simulink model "Model"  (R2024b)
settings: Solver=VariableStepAuto  StartTime=0.0  StopTime=20  RelTol=1e-2
values from neighbouring files (symbols this model uses):
  camber = 1 *pi/180    (= 0.0174532925199)    [var.m]
  cgToRearAxle = 0.7    [var.m]
  cgVerticalToAxlePlane = 0.1    [var.m]
  lammux = 0.65    [var.m]
  lammuy = 0.65    [var.m]
  mass = 200    [var.m]
  maxBrakePressure = 5000000    [var.m]
  tirePressure = 83000    [var.m]
  tireRadius = 0.2057    [var.m]
  trackWidth = 1    [var.m]
  wheelAngleLimit = 45 *pi/180    (= 0.785398163397)    [var.m]
  yawPolarInertia = 200    [var.m]
undefined symbols (not defined in the file or in its folder): SteerLim, Ts, VEH
libraries: sim3dlib x4, autolibsharedcoupling x2, sim3dautolib x2, vehdynlibviscommon x2, simulink x1, autolibshared x1, autolibshareddiff x1, autolibmappedmotor x1, vehdynlibdriver x1, vehdynlibsteering x1, vehdynlibtire x1, vehdynlibsuspension x1
(part 1 of 3)
settings Model: Creator=owen  LastModifiedBy=owen

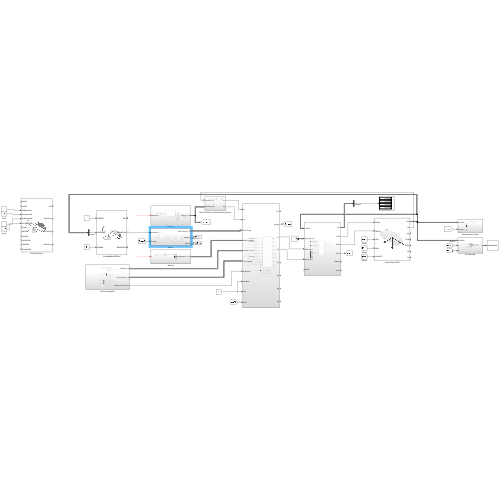
[thumbnail: Simulink's stored preview of the top-level diagram]
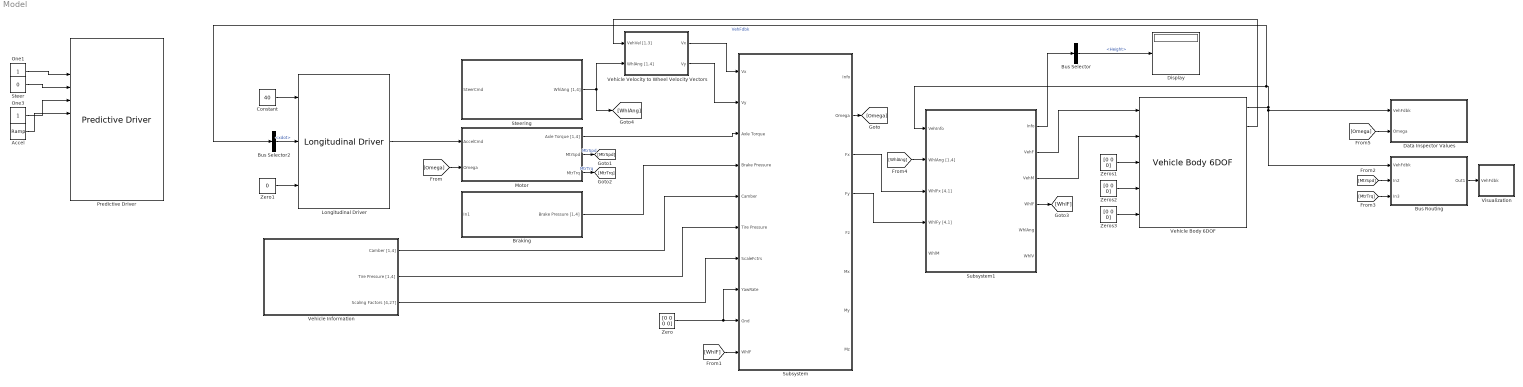
== system Model ==
  Accel : simulink/Sources/Ramp  slope=0.1  start=0  InitialOutput=0
  Braking : Subsystem
  Bus Selector : BusSelector  OutputSignals=Height
  Bus Selector2 : BusSelector  OutputSignals=BdyFrm.Cg.Vel.xdot
  Bus Routing : Subsystem
  Constant : Constant  Value=40
  Data Inspector Values : Subsystem
  Display : Display
  Longitudinal Driver : autolibshared/Longitudinal Driver  extAccelOvr=off  extDecelOvr=off  extAccelHld=off  extDecelHld=off  extAccelZero=off  extDecelZero=off  cntrlType=PI  shftType=None  velUnits=m/s  gearOut=off  Kp=10  Ki=5  Kff=.1  Kg=0  VehVelVec=[0 100]  KffVec=[.1 .1]  KpVec=[10 10]  KiVec=[5 5]  KgVec=[0 0]  m=1500  Kpt=3000  tau=.1  L=2  aR=200  bR=2.5  cR=.5  g=9.81  vnom=5  Kaw=1  tauerr=.01  tauPt=2  GearInit=0  tShift=.1  pdlVec=[0.1 0.4 0.5 0.9]  upShftTbl=[-1 12.9375 26.4375 39.9375 51.18749999999999 62.4375 72.84375 83.25;-1 16.3125 29.8125 43.3125 54.5624 65.8125 76.78125 87.75;-1 19.6875 33.1875 46.68749999999999 57.9375 69.1875 80.71875 92.25;-1 33 52.5 77.25 100.5 138.75 161.875 185]  dwnShftTbl=[1 9.5625 23.0625 36.5625 47.8125 59.0625 68.90625 78.75;1 12.9375 26.4375 39.9375 51.18749999999999 62.4375 72.84375 83.25;1 16.3125 29.8125 43.3125 54.562499 65.8125 76.78125 87.75;1 19.6875 33.1875 46.68749999999999 57.9375 69.1875 80.71875 92.25]  tClutch=.5  tRev=.5  tPark=120  aMode=2  UpGearVec="[0  1  2  3  4  5  6  7]"  DownGearVec="[1  2  3  4  5  6  7  8]"
      settings: LibrarySourceBlock=vehdynlibdriver/Longitudinal Driver
  Motor : Subsystem
  One1 : Constant  OutDataTypeStr=boolean
  One3 : Constant  OutDataTypeStr=boolean
  Predictive Driver : vehdynlibdriver/Predictive Driver  extAccelOvr=on  extDecelOvr=off  extAccelHld=off  extDecelHld=off  extAccelZero=off  extDecelZero=off  extSteerOvr=on  extSteerHld=off  extSteerZero=off  cntrlType=PI  cntrlTypeLat=Predictive  shftType=None  coordMode=SAE J670 (Z-down)  refType=Reference pose  velUnits=m/s  angUnits=rad  gearOut=off  steerOut=off  Kp=10  Ki=5  Kff=.1  Kg=0  VehVelVec=[0 100]  KffVec=[.1 .1]  KpVec=[10 10]  KiVec=[5 5]  KgVec=[0 0]  vnom=5  Kaw=1  tauerr=.01  tau=0.1  L=3  Kpt=3000  aR=200  bR=2.5  cR=.5  g=9.81  vecPose=off  dynamMode=off  PositionGainF=2.5  PositionGainR=2.5  YawRateGain=.2  DelayGain=.2  enableDrift=off  BetaRef=20*pi/180  KpBeta=1  KpDrift=2  KdDrift=1  KpPsi=6  KOmega=30  tOmega=1  a=cgToFrontAxle  b=cgToRearAxle  m=mass  Cy_f=cornerStiffness  Cy_r=cornerStiffness  I=yawPolarInertia  Ksteer=18  theta=wheelAngleLimit  Idl=3  Re=.3  lambda_mu=1  GearInit=0  tShift=.1  pdlVec=[0.1 0.4 0.5 0.9]  upShftTbl=[-1 12.9375 26.4375 39.9375 51.18749999999999 62.4375 72.84375 83.25;-1 16.3125 29.8125 43.3125 54.5624 65.8125 76.78125 87.75;-1 19.6875 33.1875 46.68749999999999 57.9375 69.1875 80.71875 92.25;-1 33 52.5 77.25 100.5 138.75 161.875 185]  dwnShftTbl=[-1 12.9375 26.4375 39.9375 51.18749999999999 62.4375 72.84375 83.25;-1 16.3125 29.8125 43.3125 54.5624 65.8125 76.78125 87.75;-1 19.6875 33.1875 46.68749999999999 57.9375 69.1875 80.71875 92.25;-1 33 52.5 77.25 100.5 138.75 161.875 185]  tClutch=.5  tRev=.5  tPark=120  UpGearVec="[0  1  2  3  4  5  6  7]"  DownGearVec="[1  2  3  4  5  6  7  8]"  aMode=2
  Steer : Constant  Value=0  OutDataTypeStr=Inherit: Inherit via back propagation
  Steering : Subsystem
  Subsystem : Subsystem
  Subsystem1 : Subsystem
  Vehicle Body 6DOF : vehdynlibeom/Vehicle Body 6DOF  extPos=on  extVel=on  extEuler=on  extRotRate=on  htchFMode=off  htchMMode=off  m=mass  a=cgToFrontAxle  b=cgToRearAxle  d=0  h=cgVerticalToAxlePlane  dh=1  hl=0  hh=0.1  Xe_o=[0,0, -0.25]  xbdot_o=[0,0,0]  eul_o=[0,0,0]  p_o=[0,0,0]  Iveh=[430 0 0; 0 1900 0; 0 0 2100]  w=[trackWidth,trackWidth]  z1m=0  z1R=[-.25,.125,.15]  z1I=[1.4,-.2,.1;-.2,1.4,.1;.1,.1,2.25].*0  z2m=0  z2R=[1.4,0,.8]  z2I=[1.4,-.2,.1;-.2,1.4,.1;.1,.1,2.25].*0  z3m=0  z3R=[.75,-.5,.4]  z3I=[5,-.1,-2;-2,9,.1;-.1,.1,6].*0  z4m=0  z4R=[.75,.5,.4]  z4I=[5,-.1,-2;-2,9,.1;-.1,.1,6].*0  z5m=0  z5R=[1.25,-.5,.4]  z5I=[5,-.1,-2;-2,9,.1;-.1,.1,6].*0  z6m=0  z6R=[1.25,-.5,.4]  z6I=[5,-.1,-2;-2,9,.1;-.1,.1,6].*0  z7m=0  z7R=[2,0,.25]  z7I=[1.4,-.2,.1;-.2,1.4,.1;.1,.1,2.25].*0  Af=longDragArea  Cd=longDragCoeff  Cl=longLiftCoeff  Cpm=.1  beta_w=[0:0.001:0.01]  Cs=[0:0.01:0.1]  Cym=[0:0.001:0.01]  Pabs=101325  extTamb=off  Tair=273  g=9.81  xdot_tol=.1  longOff=0  latOff=0  vertOff=0  wrapAng=on  aMode=2
  Vehicle Information : Subsystem
  Vehicle Velocity to Wheel Velocity Vectors : Subsystem
  Visualization : Subsystem
      mask Display: disp('Visualization')
  Zero : Constant  Value=[0 0 0 0]
  Zero1 : Constant  Value=0  OutDataTypeStr=Inherit: Inherit via back propagation
  Zeros1 : Constant  Value=[0 0 0]
  Zeros2 : Constant  Value=[0 0 0]
  Zeros3 : Constant  Value=[0 0 0]
  wires:
  ? -> Steering/1(SteerCmd)
  Steer/1 -> Predictive Driver/4
  One1/1 -> Predictive Driver/3
  Longitudinal Driver/2 -> Motor/1(AccelCmd)
  ? -> Braking/1(In1)
  Braking/1("Brake Pressure [1,4] ") -> Subsystem/4(Brake Pressure)
  Motor/1(Axle Torque [1,4]) -> Subsystem/3(Axle Torque)
  Vehicle Information/1(Camber [1,4]) -> Subsystem/5(Camber)
  Vehicle Information/2(Tire Pressure [1,4]) -> Subsystem/6(Tire Pressure)
  Vehicle Body 6DOF/2 -> Vehicle Velocity to Wheel Velocity Vectors/1(VehVel [1,3])
  Steering/1(WhlAng [1,4]) -> [WhlAng], Vehicle Velocity to Wheel Velocity Vectors/2(WhlAng [1,4])
  Vehicle Velocity to Wheel Velocity Vectors/2(Vy) -> Subsystem/2(Vy)
  Vehicle Velocity to Wheel Velocity Vectors/1(Vx) -> Subsystem/1(Vx)
  Vehicle Information/3(Scaling Factors [4,27]) -> Subsystem/7(ScaleFctrs)
  Subsystem/3(Fx) -> Subsystem1/3(WhlFx [4,1])
  Subsystem/4(Fy) -> Subsystem1/4(WhlFy [4,1])
  Subsystem1/2(VehF) -> Vehicle Body 6DOF/1
  Subsystem1/3(VehM) -> Vehicle Body 6DOF/2
  Zeros2/1 -> Vehicle Body 6DOF/4
  Zero/1 -> Subsystem/8(YawRate), Subsystem/9(Gnd)
  Vehicle Body 6DOF/1 -> Bus Routing/1(VehFdbk), Data Inspector Values/1(VehFdbk), Bus Selector2/1, Subsystem1/1(VehInfo)  "VehFdbk"
  Subsystem1/1(Info) -> Bus Selector/1
  Bus Selector/1 -> Display/1  "<Height>"
  Zeros1/1 -> Vehicle Body 6DOF/3
  Zeros3/1 -> Vehicle Body 6DOF/5
  One3/1 -> Predictive Driver/5
  Accel/1 -> Predictive Driver/6
  Subsystem/2(Omega) -> [Omega]
  [Omega] -> Motor/2(Omega)
  Motor/2(MtrSpd) -> [MtrSpd]  "MtrSpd"
  Motor/3(MtrTrq) -> [MtrTrq]  "MtrTrq"
  [MtrSpd] -> Bus Routing/2(In2)
  [MtrTrq] -> Bus Routing/3(In3)
  Bus Routing/1(Out1) -> Visualization/1(VehFdbk)
  Subsystem1/4(WhlF) -> [WhlF]
  [WhlF] -> Subsystem/10(WhlF)
  [WhlAng] -> Subsystem1/2(WhlAng [1,4])
  Zero1/1 -> Longitudinal Driver/3
  Bus Selector2/1 -> Longitudinal Driver/2  "<xdot>"
  Constant/1 -> Longitudinal Driver/1
  [Omega] -> Data Inspector Values/2(Omega)

== system Model/Braking ==
  In1 : Inport
  Bus Creator : BusCreator  Inputs=4
  Max Brake Pressure : Gain  Gain=maxBrakePressure
  "Brake Pressure [1,4] " : Outport
  wires:
  In1/1 -> Max Brake Pressure/1
  Max Brake Pressure/1 -> Bus Creator/4, Bus Creator/3, Bus Creator/2, Bus Creator/1
  Bus Creator/1 -> "Brake Pressure [1,4] "/1

== system Model/Bus Routing ==
  VehFdbk : Inport
  In2 : Inport  Port=2
  In3 : Inport  Port=3
  Bus Creator : BusCreator  Inputs=3
  Bus Creator1 : BusCreator  Inputs=2
  Bus Creator2 : BusCreator  Inputs=1
  Bus Selector3 : BusSelector  OutputSignals=InertFrm,BdyFrm
  Out1 : Outport
  wires:
  Bus Selector3/2 -> Bus Creator/2  "<BdyFrm>"
  Bus Creator/1 -> Bus Creator2/1  "VehFdbk"
  In3/1 -> Bus Creator1/2
  Bus Selector3/1 -> Bus Creator/1  "<InertFrm>"
  VehFdbk/1 -> Bus Selector3/1
  Bus Creator1/1 -> Bus Creator/3  "Mtr"
  Bus Creator2/1 -> Out1/1
  In2/1 -> Bus Creator1/1

== system Model/Data Inspector Values ==
  VehFdbk : Inport
  Omega : Inport  Port=2
  Add Constant : Bias  Bias=-1  SaturateOnIntegerOverflow=off
  Bus Selector1 : BusSelector  OutputSignals=InertFrm.Cg.Disp.Z
  Bus Selector2 : BusSelector  OutputSignals=BdyFrm.Cg.Acc.ax,BdyFrm.Cg.Acc.ay
  Bus Selector4 : BusSelector  OutputSignals=InertFrm.Cg.Vel.Xdot
  Constant3 : Constant  Value=0.2057
  Display1 : Display
  Display2 : Display
  Display3 : Display
  Divide : Product  Inputs=*/
  Product : Product
  Selector : Selector  InputPortWidth=4  IndexOptions=Index vector (dialog)  Indices=[3]  OutputSizes=1
  wires:
  Bus Selector2/1 -> Display2/1  "<ax>"
  Bus Selector2/2 -> Display3/1  "<ay>"
  VehFdbk/1 -> Bus Selector4/1, Bus Selector1/1, Bus Selector2/1
  Selector/1 -> Product/2
  Constant3/1 -> Product/1
  Bus Selector1/1 -> Display1/1  "<Z>"
  Product/1 -> Divide/1
  Bus Selector4/1 -> Divide/2  "<Xdot>"
  Omega/1 -> Selector/1
  Divide/1 -> Add Constant/1
  Add Constant/1 -> ?  "Slip ratio"

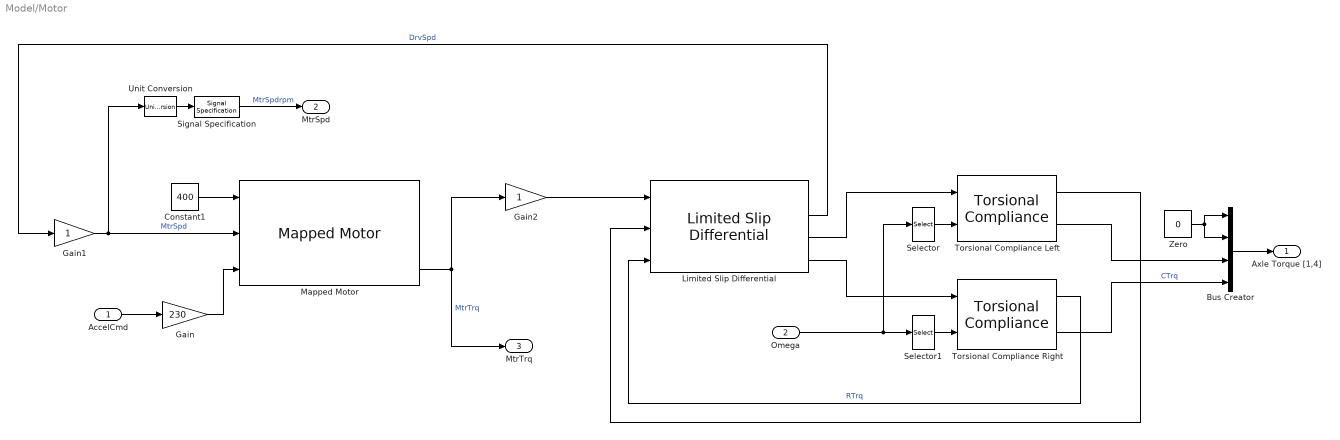
== system Model/Motor ==
  AccelCmd : Inport
  Omega : Inport  Port=2
  Bus Creator : BusCreator  Inputs=4
  Constant1 : Constant  Value=400
  Gain : Gain  Gain=230
  Gain1 : Gain
  Gain2 : Gain
  Limited Slip Differential : autolibshareddiff/Limited Slip Differential  DiffEffModelPopup=Constant  InterpMethod=Linear point-slope  extTamb=off  shaftSwitchMask=To the left of center-line  Ndiff=finalDriveRatio  Jd=.1  bd=1e-3  Jw1=.1  bw1=1e-3  Jw2=.1  bw2=1e-3  omegaw1o=0  omegaw2o=0  eta=1  eta_tbl=reshape([0.64 0.76 0.8 0.81 0.83 0.84 0.84 0.56 0.73 0.78 0.8 0.83 0.84 0.84 0.54 0.71 0.77 0.8 0.82 0.84 0.84 0.53 0.71 0.77 0.8 0.83 0.84 0.84 0.51 0.71 0.77 0.8 0.83 0.84 0.85 0.52 0.7 0.77 0.8 0.83 0.84 0.85 0.51 0.71 0.76 0.79 0.83 0.84 0.85 0.5 0.69 0.76 0.79 0.82 0.84 0.85 0.45 0.68 0.75 0.78 0.82 0.84 0.85 0.43 0.67 0.74 0.78 0.81 0.83 0.84 0.38 0.63 0.71 0.75 0.8 0.82 0.83 0.81 0.86 0.88 0.89 0.89 0.89 0.9 0.77 0.85 0.87 0.88 0.89 0.9 0.9 0.72 0.82 0.86 0.87 0.88 0.89 0.9 0.68 0.8 0.84 0.86 0.88 0.89 0.89 0.67 0.8 0.84 0.86 0.88 0.89 0.9 0.67 0.8 0.84 0.86 0.88 0.89 0.9 0.65 0.8 0.84 0.86 0.88 0.89 0.9 0.64 0.79 0.83 0.86 0.88 0.89 0.9 0.63 0.78 0.83 0.86 0.88 0.89 0.9 0.59 0.76 0.82 0.85 0.87 0.89 0.9 0.53 0.73 0.8 0.83 0.86 0.88 0.89], 7, 11, 2)  Trq_bpts=[25, 50, 75, 100, 150, 200, 250]  omega_bpts=[52.4 78.5 105 131 157 183 209 262 314 419 524]  Temp_bpts=[290 358]  Tamb=297.15  couplingType=Pre-loaded ideal clutch  Ndisks=4  Reff=.20  Fc=500  muc=[.16 0.13 0.115 0.11 0.105 0.1025 0.10125]  dw=[0 10 20 40 60 80 100]  Tdw=[-100, -90, -50, -5, 0, 5, 50, 90, 100]  dwT=[-200, -175, -100, - 50, 0, 50, 100, 175, 200]  TTin=[-200 -175 -100 - 50 0 50 100 175 200]  Tin=[-200 -175 -100 - 50 0 50 100 175 200]  tauC=.01  IdealInterpMethod=Linear point-slope  IdealExtrapMethod=Clip  TdwInterpMethod=Linear point-slope  TdwExtrapMethod=Clip  TTinInterpMethod=Linear point-slope  TTinExtrapMethod=Clip  maxAbsSpd=5e3  aMode=2
      settings: LibrarySourceBlock=vdynlib/Powertrain/Drivetrain/Final Drive Unit/Limited Slip Differential
  Mapped Motor : autolibmappedmotor/Mapped Motor  w_Tmax_bp_ext=w_Tmax_bp  Tmax_w_V_ext=Tmax_w_V  w_Tmin_bp_ext=w_Tmin_bp  Tmin_w_V_ext=Tmin_w_V  port_config=Speed  param_by=Tabulated torque-speed envelope  w_t=motorSpeedBreakpoints  T_t=motorTorqueBreakpoints  torque_max=.1  power_max=30  SpreadsheetTqLimitsFileName=MotorCalibrationImportData.xlsx  Tmax_w_V=[0.09 0.09 0.09;0.08 0.08 0.08;0.07 0.07 0.07;0 0 0]  w_Tmax_bp=[ 0 375 750 800 ]  V_Tmax_bp=[500 750 900]  Tmin_w_V=[-0.09 -0.09 -0.09;-0.08 -0.08 -0.08;-0.07 -0.07 -0.07;0 0 0]  w_Tmin_bp=[ 0 375 750 800 ]  V_Tmin_bp=[500 750 900]  Tc=torqueControlTimeConstant  param_loss=Single efficiency measurement  SpreadsheetLossFileName=MotorCalibrationImportData.xlsx  SpreadsheetEffFileName=MotorCalibrationImportData.xlsx  eff=100  w_eff=375  T_eff=0.08  Piron=0  Pbase=0  w_eff_bp=[-800 -400 0 400 800]  T_eff_bp=[0 0.03 0.06 0.09]  Temp_eff_bp=[233.15 293.15 373.15]  V_eff_bp=[500 700 900]  losses_table=[1.49 1.67 2.21 3.10; 0.42 0.69 1.14 2.03; 0.06 0.24 0.78 1.68; 0.42 0.69 1.14 2.03; 1.49 1.67 2.21 3.10]  losses_table_3d=cat(3,[1.49 1.67 2.21 3.10; 0.42 0.69 1.14 2.03; 0.06 0.24 0.78 1.68; 0.42 0.69 1.14 2.03; 1.49 1.67 2.21 3.10],[1.49 1.67 2.21 3.10; 0.42 0.69 1.14 2.03; 0.06 0.24 0.78 1.68; 0.42 0.69 1.14 2.03; 1.49 1.67 2.21 3.10],[1.49 1.67 2.21 3.10; 0.42 0.69 1.14 2.03; 0.06 0.24 0.78 1.68; 0.42 0.69 1.14 2.03; 1.49 1.67 2.21 3.10])  losses_table_4d=cat(4,cat(3,[1.5645 0.441 0.063 0.441 1.5645;1.7535 0.7245 0.252 0.7245 1.7535;2.3205 1.197 0.819 1.197 2.3205;3.255 2.1315 1.764 2.1315 3.255],[1.5645 0.441 0.063 0.441 1.5645;1.7535 0.7245 0.252 0.7245 1.7535;2.3205 1.197 0.819 1.197 2.3205;3.255 2.1315 1.764 2.1315 3.255],[1.5645 0.441 0.063 0.441 1.5645;1.7535 0.7245 0.252 0.7245 1.7535;2.3205 1.197 0.819 1.197 2.3205;3.255 2.1315 1.764 2.1315 3.255]),cat(3,[1.49 0.42 0.06 0.42 1.49;1.67 0.69 0.24 0.69 1.67;2.21 1.14 0.78 1.14 2.21;3.1 2.03 1.68 2.03 3.1],[1.49 0.42 0.06 0.42 1.49;1.67 0.69 0.24 0.69 1.67;2.21 1.14 0.78 1.14 2.21;3.1 2.03 1.68 2.03 3.1],[1.49 0.42 0.06 0.42 1.49;1.67 0.69 0.24 0.69 1.67;2.21 1.14 0.78 1.14 2.21;3.1 2.03 1.68 2.03 3.1]),cat(3,[1.5347 0.4326 0.0618 0.4326 1.5347;1.7201 0.7107 0.2472 0.7107 1.7201;2.2763 1.1742 0.8034 1.1742 2.2763;3.193 2.0909 1.7304 2.0909 3.193],[1.5347 0.4326 0.0618 0.4326 1.5347;1.7201 0.7107 0.2472 0.7107 1.7201;2.2763 1.1742 0.8034 1.1742 2.2763;3.193 2.0909 1.7304 2.0909 3.193],[1.5347 0.4326 0.0618 0.4326 1.5347;1.7201 0.7107 0.2472 0.7107 1.7201;2.2763 1.1742 0.8034 1.1742 2.2763;3.193 2.0909 1.7304 2.0909 3.193]))  efficiency_table=[95 95 95 95; 95 95 95 95; 95 95 95 95; 95 95 95 95; 95 95 95 95]  efficiency_table_3d=cat(3,[95 95 95 95; 95 95 95 95; 95 95 95 95; 95 95 95 95; 95 95 95 95],[95 95 95 95; 95 95 95 95; 95 95 95 95; 95 95 95 95; 95 95 95 95],[95 95 95 95; 95 95 95 95; 95 95 95 95; 95 95 95 95; 95 95 95 95])  efficiency_table_4d=cat(4,cat(3,90*ones(5,4)',90*ones(5,4)',90*ones(5,4)'),cat(3,95*ones(5,4)',95*ones(5,4)',95*ones(5,4)'),cat(3,92*ones(5,4)',92*ones(5,4)',92*ones(5,4)'))  J=5e-6  b=1e-5  omega_o=0  T_t_extended=[0 175 230 230 220 230 230 175 0]  w_t_extended=[-680.783128032908 -680.678408277789 -523.598775598299 -52.3598775598299 0 52.3598775598299 523.598775598299 680.678408277789 680.783128032908]  KLossIron=0  KLossCopper=0  x_w_eff_vec=[-8000 -4000 0 4000 8000]  x_T_eff_vec=[-0.09 -0.06 -0.03 0 0.03 0.06 0.09]  x_tmp_eff_vec=[-0.09 -0.06 -0.03 0 0.03 0.06 0.09]  x_V_eff_vec=[500 700 900]  x_losses_mat=[3.1 2.21 1.67 1.49 1.67 2.21 3.1;2.03 1.14 0.69 0.42 0.69 1.14 2.03;1.68 0.78 0.24 0.06 0.24 0.78 1.68;2.03 1.14 0.69 0.42 0.69 1.14 2.03;3.1 2.21 1.67 1.49 1.67 2.21 3.1]  x_losses_mat_3d=[37.8947368421052 25.2631578947368 12.6315789473684 0 12 24 36;18.9473684210526 12.6315789473684 6.3157894736842 0 5.99999999999999 12 18;0 0 0 0 0 0 0;18 12 5.99999999999999 0 6.3157894736842 12.6315789473684 18.9473684210526;36 24 12 0 12.6315789473684 25.2631578947368 37.8947368421052]  x_losses_mat_4d=cat(4,cat(3,[1.5645 0.441 0.063 0.441 1.5645;1.7535 0.7245 0.252 0.7245 1.7535;2.3205 1.197 0.819 1.197 2.3205;3.255 2.1315 1.764 2.1315 3.255],[1.5645 0.441 0.063 0.441 1.5645;1.7535 0.7245 0.252 0.7245 1.7535;2.3205 1.197 0.819 1.197 2.3205;3.255 2.1315 1.764 2.1315 3.255],[1.5645 0.441 0.063 0.441 1.5645;1.7535 0.7245 0.252 0.7245 1.7535;2.3205 1.197 0.819 1.197 2.3205;3.255 2.1315 1.764 2.1315 3.255]),cat(3,[1.49 0.42 0.06 0.42 1.49;1.67 0.69 0.24 0.69 1.67;2.21 1.14 0.78 1.14 2.21;3.1 2.03 1.68 2.03 3.1],[1.49 0.42 0.06 0.42 1.49;1.67 0.69 0.24 0.69 1.67;2.21 1.14 0.78 1.14 2.21;3.1 2.03 1.68 2.03 3.1],[1.49 0.42 0.06 0.42 1.49;1.67 0.69 0.24 0.69 1.67;2.21 1.14 0.78 1.14 2.21;3.1 2.03 1.68 2.03 3.1]),cat(3,[1.5347 0.4326 0.0618 0.4326 1.5347;1.7201 0.7107 0.2472 0.7107 1.7201;2.2763 1.1742 0.8034 1.1742 2.2763;3.193 2.0909 1.7304 2.0909 3.193],[1.5347 0.4326 0.0618 0.4326 1.5347;1.7201 0.7107 0.2472 0.7107 1.7201;2.2763 1.1742 0.8034 1.1742 2.2763;3.193 2.0909 1.7304 2.0909 3.193],[1.5347 0.4326 0.0618 0.4326 1.5347;1.7201 0.7107 0.2472 0.7107 1.7201;2.2763 1.1742 0.8034 1.1742 2.2763;3.193 2.0909 1.7304 2.0909 3.193]))  CalLossMapData={}  CalLossWithTempMapData={}  aMode=1  RefBlkName='autolibmappedmotor/Mapped Motor'
      settings: LibrarySourceBlock=autolibemachines/Mapped Motor
  Selector : Selector  InputPortWidth=4  IndexOptions=Index vector (dialog)  Indices=[3]  OutputSizes=1
  Selector1 : Selector  InputPortWidth=4  IndexOptions=Index vector (dialog)  Indices=[4]  OutputSizes=1
  Signal Specification : SignalSpecification  Unit=rpm
  Torsional Compliance Left : autolibsharedcoupling/Torsional Compliance  port_config=Simulink  extInfo=off  k=1e4  b=1e2  theta_o=0  domega_o=0  omega_c=3000  blkID=0  aMode=2
      settings: LibrarySourceBlock=vdynlib/Powertrain/Drivetrain/Couplings/Torsional Compliance
  Torsional Compliance Right : autolibsharedcoupling/Torsional Compliance  port_config=Simulink  extInfo=off  k=1e4  b=1e2  theta_o=0  domega_o=0  omega_c=3000  blkID=0  aMode=2
      settings: LibrarySourceBlock=vdynlib/Powertrain/Drivetrain/Couplings/Torsional Compliance
  Unit Conversion : UnitConversion
  Zero : Constant  Value=0  OutDataTypeStr=Inherit: Inherit via back propagation
  Axle Torque [1,4] : Outport
  MtrSpd : Outport  Port=2
  MtrTrq : Outport  Port=3
  wires:
  Bus Creator/1 -> Axle Torque [1,4]/1
  Zero/1 -> Bus Creator/1, Bus Creator/2
  Gain/1 -> Mapped Motor/3
  Constant1/1 -> Mapped Motor/1
  AccelCmd/1 -> Gain/1
  Mapped Motor/3 -> Gain2/1, MtrTrq/1  "MtrTrq"
  Limited Slip Differential/3 -> Torsional Compliance Left/1
  Limited Slip Differential/4 -> Torsional Compliance Right/1
  Omega/1 -> Selector/1, Selector1/1
  Selector1/1 -> Torsional Compliance Right/2
  Selector/1 -> Torsional Compliance Left/2
  Torsional Compliance Left/2 -> Bus Creator/3
  Torsional Compliance Right/2 -> Bus Creator/4  "CTrq"
  Torsional Compliance Left/1 -> Limited Slip Differential/2
  Torsional Compliance Right/1 -> Limited Slip Differential/3  "RTrq"
  Limited Slip Differential/2 -> Gain1/1  "DrvSpd"
  Unit Conversion/1 -> Signal Specification/1
  Signal Specification/1 -> MtrSpd/1  "MtrSpdrpm"
  Gain1/1 -> Unit Conversion/1, Mapped Motor/2  "MtrSpd"
  Gain2/1 -> Limited Slip Differential/1

== system Model/Steering ==
  SteerCmd : Inport
  Bus Creator : BusCreator  Inputs=4
  Gain : Gain  Gain=wheelAngleLimit
  Kinematic Steering : vehdynlibsteering/Kinematic Steering  StrgType=Ackerman  StrgRatioType=Constant  Loc=Front  NrmlFctr=1  TrckWdth=trackWidth  WhlBase=wheelBase  Db=0  StrgRng=wheelAngleLimit  StrgAngBpts="[-6.2832   -5.0265   -3.7699   -2.5133   -1.2566         0    1.2566    2.5133    3.7699    5.0265    6.2832]"  StrgRatioTbl=|  StrgRatio=1  PctAckIn=off  PctAck=100  PctAckTbl=ones(1,11)*100  StrgArmLngth=0.1  RckCsLngth=0.5  TieRodLngth=0.248  D=0.2  PnnRadius=0.00085818  PnnRadiusTbl="[0.0055    0.0055    0.0056    0.0057    0.0058    0.0057    0.0057    0.0057    0.0056    0.0055    0.0055]"  RodLngth=0.1  ParaArmLngth=0.9  aMode=2
      | [13.5000   13.3750   13.2500   13.1250   13.0000   13.0000   13.0000   13.1250   13.2500   13.3750   13.5000
      | ]
  Zero : Constant  Value=0  OutDataTypeStr=Inherit: Inherit via back propagation
  WhlAng [1,4] : Outport
  wires:
  Gain/1 -> Kinematic Steering/1
  SteerCmd/1 -> Gain/1
  Kinematic Steering/2 -> Bus Creator/1
  Kinematic Steering/3 -> Bus Creator/2
  Zero/1 -> Bus Creator/4, Bus Creator/3
  Bus Creator/1 -> WhlAng [1,4]/1

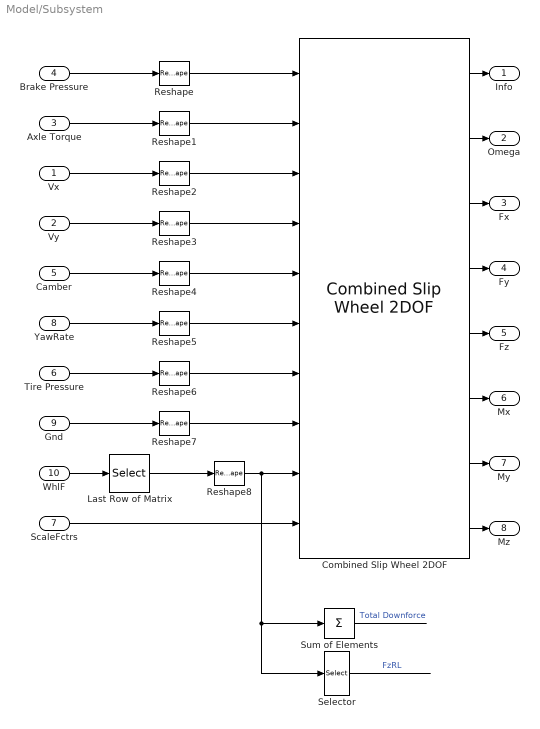
== system Model/Subsystem ==
  Vx : Inport
  Vy : Inport  Port=2
  Axle Torque : Inport  Port=3
  Brake Pressure : Inport  Port=4
  Camber : Inport  Port=5
  Tire Pressure : Inport  Port=6
  ScaleFctrs : Inport  Port=7
  YawRate : Inport  Port=8
  Gnd : Inport  Port=9
  WhlF : Inport  Port=10
  Combined Slip Wheel 2DOF : vehdynlibtire/Combined Slip Wheel 2DOF  tireType=External file  tireParamSet=C:\Users\owen\MATLAB\Projects\Vehicle Model New\Fx 16x7.5-10-7.tir  vertType=Magic Formula  plySteer=off  turnslip=off  BrakeType=Disc  mu_static=staticFriction  mu_kinetic=kineticFriction  drum_abore=0.0508  drum_a=0.123  drum_c=0.212  drum_r=0.15  drum_theta1=0  drum_theta2=126  disk_abore=discBrakeActuatorBore  Rm=brakePadMeanRadius  num_pads=numBrakePads  brake_p_bpt=[1 11.4736842105263 21.9473684210526 32.4210526315789 42.8947368421053 53.3684210526316 63.8421052631579 74.3157894736842 84.7894736842105 95.2631578947368 105.736842105263 116.210526315789 126.684210526316 137.157894736842 147.631578947368 158.105263157895 168.578947368421 179.052631578947 189.526315789474 200]  brake_n_bpt=[0 52.6315789473684 105.263157894737 157.894736842105 210.526315789474 263.157894736842 315.789473684211 368.421052631579 421.052631578947 473.684210526316 526.315789473684 578.947368421053 631.578947368421 684.210526315789 736.842105263158 789.473684210526 842.105263157895 894.736842105263 947.368421052632 1000]  f_brake_t=[43.4900602404453 42.5056030554862 41.5350898940194 40.5780454442085 39.6340111501808 38.7025443887544 37.7832176914519 36.8756180088306 35.9793460143796 35.0940154454303 34.2192524787115 33.3546951383474 32.4999927342521 31.6548053290159 30.8188032315107 29.991666515561 29.1730845621415 28.362755623661 27.5603864089927 26.765691687993;498.991217495636 487.695866636631 476.560505099801 465.579679307235 454.748127933653 444.060772460445 433.51270824929 423.099196101319 412.81565427025 402.657650900201 392.620896861006 382.701238955775 372.894653477208 363.197240090814 353.605216024701 344.114910546964 334.722759712992 325.425301366216 316.219170376863 307.10109410434;954.492374750826 932.886130217776 911.585920305583 890.581313170261 869.862244717126 849.419000532136 829.242198807128 809.322774193808 789.651962526121 770.221286354971 751.0225412433 732.047782773203 713.289314220164 694.739674852612 676.391628817892 658.238154578366 640.272434863842 622.48784710877 604.877954344734 587.436496520688;1409.99353200602 1378.07639379892 1346.61133551136 1315.58294703329 1284.9763615006 1254.77722860383 1224.97168936497 1195.5463522863 1166.48827078199 1137.78492180974 1109.42418562559 1081.39432659063 1053.68397496312 1026.28210961441 999.178041611083 972.361398609768 945.822110014692 919.550392851325 893.536738312604 867.771898937035;1865.49468926121 1823.26665738007 1781.63675071715 1740.58458089631 1700.09047828407 1660.13545667552 1620.7011799228 1581.76993037878 1543.32457903786 1505.34855726451 1467.82583000789 1430.74087040806 1394.07863570608 1357.82454437621 1321.96445440427 1286.48464264117 1251.37178516554 1216.61293859388 1182.19552228048 1148.10730135338;2320.9958465164 2268.45692096121 2216.66216592293 2165.58621475934 2115.20459506754 2065.49368474721 2016.43067048064 1967.99350847127 1920.16088729373 1872.91219271928 1826.22747439018 1780.08741422549 1734.47329644903 1689.36697913801 1644.75086719747 1600.60788667257 1556.92146031639 1513.67548433643 1470.85430624835 1428.44270376973;2776.49700377159 2713.64718454235 2651.68758112871 2590.58784862237 2530.31871185102 2470.8519128189 2412.16016103848 2354.21708656376 2296.9971955496 2240.47582817405 2184.62911877248 2129.43395804292 2074.86795719199 2020.9094138998 1967.53727999066 1914.73113070398 1862.47113546724 1810.73803007899 1759.51309021622 1708.77810618608;3231.99816102678 3158.8374481235 3086.71299633449 3015.58948248539 2945.43282863449 2876.21014089059 2807.88965159632 2740.44066465625 2673.83350380547 2608.03946362882 2543.03076315477 2478.78050186034 2415.26261793494 2352.4518486616 2290.32369278385 2228.85437473538 2168.02081061809 2107.80057582154 2048.17187418409 1989.11350860242;3687.49931828197 3604.02771170464 3521.73841154027 3440.59111634842 3360.54694541796 3281.56836896228 3203.61914215416 3126.66424274874 3050.66981206134 2975.60309908359 2901.43240753707 2828.12704567777 2755.6572786779 2683.9942834234 2613.11010557704 2542.97761876678 2473.57048576894 2404.8631215641 2336.83065815196 2269.44891101877;4143.00047553716 4049.21797528579 3956.76382674606 3865.59275021144 3775.66106220143 3686.92659703397 3599.34863271199 3512.88782084123 3427.50612031721 3343.16673453836 3259.83405191936 3177.4735894952 3096.05193942085 3015.5367181852 2935.89651837023 2857.10086279818 2779.12016091979 2701.92566730665 2625.48944211983 2549.78431343512;4598.50163279235 4494.40823886693 4391.78924195184 4290.59438407447 4190.77517898491 4092.28482510566 3995.07812326983 3899.11139893372 3804.34242857308 3710.73036999313 3618.23569630166 3526.82013331263 3436.44660016381 3347.079152947 3258.68293116342 3171.22410682959 3084.66983607064 2998.98821304921 2914.1482260877 2830.11971585147;5054.00279004754 4939.59850244808 4826.81465715762 4715.59601793749 4605.88929576838 4497.64305317735 4390.80761382767 4285.3349770262 4181.17873682896 4078.2940054479 3976.63734068395 3876.16667713006 3776.84126090677 3678.62158770879 3581.46934395661 3485.34735086099 ...(+2764 chars)]  NOMPRES=83000  PRESMAX=413685.6  PRESMIN=0  FNOMIN=1110  FZMAX=100000  FZMIN=0  VXLOW=1  KPUMAX=0.99  KPUMIN=-0.99  ALPMAX=0.523598775598299  ALPMIN=-0.523598775598299  CAMMAX=0.174532925199433  CAMMIN=-0.174532925199433  LONGVL=10  FxRelFreqLwrLim=200*pi  FyRelFreqLwrLim=200*pi  MyRelFreqLwrLim=100*pi  omegao=0  UNLOADED_RADIUS=0.2057  WIDTH=0.21336  RIM_RADIUS=0.1016  ASPECT_RATIO=0.45  MASS=3.62  IYY=1.084  br=1e-3  GRAVITY=-9.81  zo=0  zdoto=0  BREFF=8.39  DREFF=0.31475  FREFF=0.14694  Q_RE0=1.003  Q_V1=0.000864  Q_V2=0.025807  Q_FZ1=0  Q_FZ2=51.51  Q_FZ3=0  Q_FCX=0  Q_FCY=0  Q_FCY2=0  PFZ1=1  VERTICAL_STIFFNESS=283576.3  VERTICAL_DAMPING=500  BOTTOM_OFFST=0.01  BOTTOM_STIFF=2000000  Q_CAM1=0  Q_CAM2=0  Q_CAM3=0  Q_FYS1=0  Q_FYS2=0  Q_FYS3=0  LONGITUDINAL_STIFFNESS=505632.6  LATERAL_STIFFNESS=219162.7  PCFX1=-0.12193  PCFX2=0  PCFX3=0  PCFY1=-0.17034  PCFY2=0  PCFY3=0  Q_RA1=0.602  Q_RA2=1.024  Q_RB1=1.1137  Q_RB2=-0.09748  PCX1=1.5154  PDX1=1.198  PDX2=-0.06303  PDX3=0  PEX1=0.3078  PEX2=-0.4082  PEX3=0  PEX4=0.05178  PKX1=45.95  PKX2=15  PKX3=-0.192  PHX1=-0.001311  PHX2=0.0005846  PVX1=0.05705  PVX2=-0.0128  PPX1=0  PPX2=0  PPX3=0  PPX4=0  RBX1=28.37  RBX2=23.625  RBX3=0  RCX1=1.0135  REX1=-0.11366  REX2=0.011092  RHX1=0.002996  QSX1=0  QSX2=1.5  QSX3=0.1  QSX4=0.1  QSX5=0  QSX6=0  QSX7=0.1  QSX8=0  QSX9=0  QSX10=0  QSX11=0  QSX12=0  QSX13=0  QSX14=0  PPMX1=0  PCY1=1.5  PDY1=2.3155  PDY2=-0.41775  PDY3=10  PEY1=-0.077579  PEY2=-0.096166  PEY3=-1.8215  PEY4=195.2442  PEY5=628.6612  PKY1=-31.141  PKY2=1.2778  PKY3=1  PKY4=2  PKY5=17.6662  PKY6=-4.7027  PKY7=-0.28572  PHY1=0.0025009  PHY2=0.0021823  PVY1=0.084054  PVY2=0.064236  PVY3=-1.7944  PVY4=0.59568  PPY1=0.49443  PPY2=1.4125  PPY3=-0.94338  PPY4=-2  PPY5=0.037053  RBY1=5  RBY2=2  RBY3=0.02  RBY4=0  RCY1=1  REY1=-0.1  REY2=0.1  RHY1=0  RHY2=0  RVY1=0  RVY2=0  RVY3=0  RVY4=0  RVY5=0  RVY6=0  QSY1=0  QSY2=0  QSY3=0  QSY4=0  QSY5=0  QSY6=0  QSY7=0  QSY8=0  QBZ1=2.2204e-16  QBZ2=0  QBZ3=0  QBZ4=0  QBZ5=0  QBZ6=0  QBZ9=0  QBZ10=0  QCZ1=0.1  QDZ1=0.1  QDZ2=0  QDZ3=0  QDZ4=0  QDZ6=0  QDZ7=0  QDZ8=0  QDZ9=0  QDZ10=0  QDZ11=0  QEZ1=0  QEZ2=0  QEZ3=0  QEZ4=0  QEZ5=0  QHZ1=0  QHZ2=0  QHZ3=0  QHZ4=0  PPZ1=0  PPZ2=0  SSZ1=0  SSZ2=0  SSZ3=0  SSZ4=0  PDXP1=0  PDXP2=0  PDXP3=0  PKYP1=0  PDYP1=0  PDYP2=0  PDYP3=0  PDYP4=0  PHYP1=0  PHYP2=0  PHYP3=0  PHYP4=0  PECP1=0  PECP2=0  QDTP1=0  QCRP1=0  QCRP2=0  QBRP1=0  QDRP1=0  QDRP2=0  aMode=2
  Last Row of Matrix : Selector  NumberOfDimensions=2  InputPortWidth=3  IndexOptions=Index vector (dialog),Select all  Indices=[3],1  OutputSizes=1,1
  Reshape{,1..8} (9 alike) : Reshape  OutputDimensionality=Column vector (2-D)
  Selector : Selector  InputPortWidth=4  IndexOptions=Index vector (dialog)  Indices=[3]  OutputSizes=1
  Sum of Elements : Sum  Inputs=+
  Info : Outport
  Omega : Outport  Port=2
  Fx : Outport  Port=3
  Fy : Outport  Port=4
  Fz : Outport  Port=5
  Mx : Outport  Port=6
  My : Outport  Port=7
  Mz : Outport  Port=8
  wires:
  Combined Slip Wheel 2DOF/6 -> Mx/1
  Combined Slip Wheel 2DOF/3 -> Fx/1
  Combined Slip Wheel 2DOF/5 -> Fz/1
  Combined Slip Wheel 2DOF/1 -> Info/1
  Combined Slip Wheel 2DOF/8 -> Mz/1
  Combined Slip Wheel 2DOF/4 -> Fy/1
  Combined Slip Wheel 2DOF/7 -> My/1
  Combined Slip Wheel 2DOF/2 -> Omega/1
  Tire Pressure/1 -> Reshape6/1
  Axle Torque/1 -> Reshape1/1
  Brake Pressure/1 -> Reshape/1
  WhlF/1 -> Last Row of Matrix/1
  Gnd/1 -> Reshape7/1
  YawRate/1 -> Reshape5/1
  Camber/1 -> Reshape4/1
  Vy/1 -> Reshape3/1
  Vx/1 -> Reshape2/1
  ScaleFctrs/1 -> Combined Slip Wheel 2DOF/10
  Reshape/1 -> Combined Slip Wheel 2DOF/1
  Reshape1/1 -> Combined Slip Wheel 2DOF/2
  Reshape2/1 -> Combined Slip Wheel 2DOF/3
  Reshape3/1 -> Combined Slip Wheel 2DOF/4
  Reshape4/1 -> Combined Slip Wheel 2DOF/5
  Reshape5/1 -> Combined Slip Wheel 2DOF/6
  Reshape6/1 -> Combined Slip Wheel 2DOF/7
  Reshape7/1 -> Combined Slip Wheel 2DOF/8
  Reshape8/1 -> Selector/1, Sum of Elements/1, Combined Slip Wheel 2DOF/9
  Last Row of Matrix/1 -> Reshape8/1
  Sum of Elements/1 -> ?  "Total Downforce"
  Selector/1 -> ?  "FzRL"

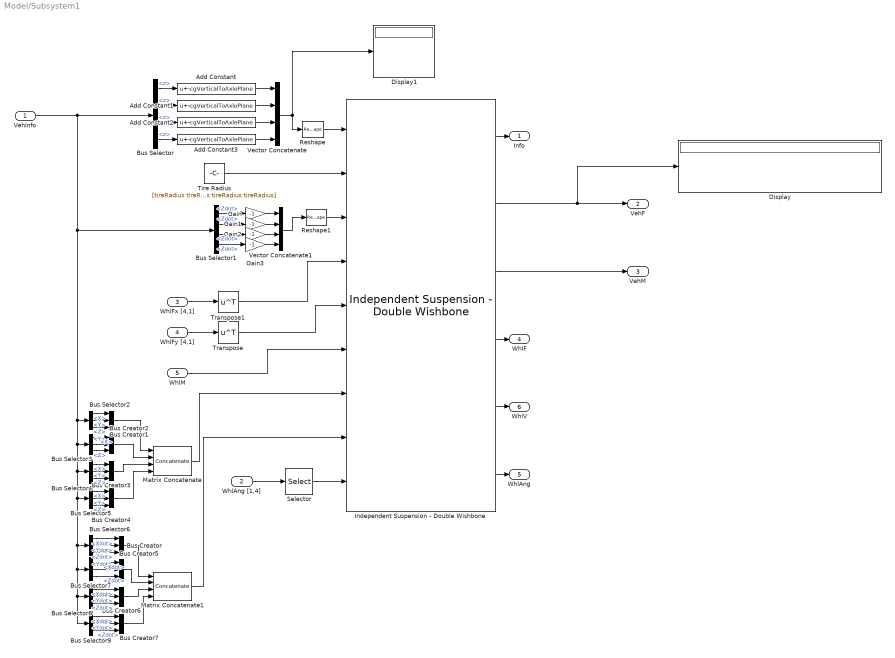
== system Model/Subsystem1 ==
  VehInfo : Inport
  WhlAng [1,4] : Inport  Port=2
  WhlFx [4,1] : Inport  Port=3
  WhlFy [4,1] : Inport  Port=4
  WhlM : Inport  Port=5
  Add Constant{,1..3} (4 alike) : Bias  Bias=-cgVerticalToAxlePlane  SaturateOnIntegerOverflow=off
  Bus Creator{,1..7} (8 alike) : BusCreator  Inputs=3
  Bus Selector : BusSelector  OutputSignals=BdyFrm.FrntAxl.Lft.Disp.z,BdyFrm.FrntAxl.Rght.Disp.z,BdyFrm.RearAxl.Lft.Disp.z,BdyFrm.RearAxl.Rght.Disp.z
  Bus Selector1 : BusSelector  OutputSignals=InertFrm.FrntAxl.Lft.Vel.Zdot,InertFrm.FrntAxl.Rght.Vel.Zdot,InertFrm.RearAxl.Lft.Vel.Zdot,InertFrm.RearAxl.Rght.Vel.Zdot
  Bus Selector2 : BusSelector  OutputSignals=InertFrm.FrntAxl.Lft.Disp.X,InertFrm.FrntAxl.Lft.Disp.Y,InertFrm.FrntAxl.Lft.Disp.Z
  Bus Selector3 : BusSelector  OutputSignals=InertFrm.FrntAxl.Rght.Disp.X,InertFrm.FrntAxl.Rght.Disp.Y,InertFrm.FrntAxl.Rght.Disp.Z
  Bus Selector4 : BusSelector  OutputSignals=InertFrm.RearAxl.Lft.Disp.X,InertFrm.RearAxl.Lft.Disp.Y,InertFrm.RearAxl.Lft.Disp.Z
  Bus Selector5 : BusSelector  OutputSignals=InertFrm.RearAxl.Rght.Disp.X,InertFrm.RearAxl.Rght.Disp.Y,InertFrm.RearAxl.Rght.Disp.Z
  Bus Selector6 : BusSelector  OutputSignals=InertFrm.FrntAxl.Rght.Vel.Xdot,InertFrm.FrntAxl.Rght.Vel.Ydot,InertFrm.FrntAxl.Rght.Vel.Zdot
  Bus Selector7 : BusSelector  OutputSignals=InertFrm.FrntAxl.Lft.Vel.Xdot,InertFrm.FrntAxl.Lft.Vel.Ydot,InertFrm.FrntAxl.Lft.Vel.Zdot
  Bus Selector8 : BusSelector  OutputSignals=InertFrm.RearAxl.Lft.Vel.Xdot,InertFrm.RearAxl.Lft.Vel.Ydot,InertFrm.RearAxl.Lft.Vel.Zdot
  Bus Selector9 : BusSelector  OutputSignals=InertFrm.RearAxl.Rght.Vel.Xdot,InertFrm.RearAxl.Rght.Vel.Ydot,InertFrm.RearAxl.Rght.Vel.Zdot
  Display : Display
  Display1 : Display
  Gain{,1..3} (4 alike) : Gain  Gain=-1
  Independent Suspension - Double Wishbone : vehdynlibsuspension/Independent Suspension - Double Wishbone  ActiveDampEn=off  NumAxl=2  NumWhlsByAxl=[2 2]  StrgEnByAxl=[1 0]  AntiSwayEnByAxl=[0 0]  WhlNumVec="[1  2  1  2]"  AxleNumVec="[1  1  2  2]"  SuspTypesByAxle="[1  1]"  SuspImage=suspdw.png  IdealSuspEn=on  IdealSuspAxles="[1  2]"  Kz=64370  F0z=9810  Cz=10000  Hmax=0.5  f_act_susp_cz=[10000 10000;10000 10000]  f_act_susp_duty_bpt=[0 1]  f_act_susp_zdot_bpt=[-1 1]  Toe=0.0349  RollStrgSlp=-0.2269  ToeStrgSlp=0.01  Caster=0.0698  CasterHslp=-0.2269  CasterStrgSlp=0.01  Camber=0.0698  CamberHslp=-0.2269  CamberStrgSlp=0.01  StrgHgtSlp=0.1432  MappedSuspEn=off  MappedSuspAxles="[1  2]"  f_susp_axl_bp=[1 2]  f_susp_dz_bp=[-0.15 -0.14 -0.13 -0.12 -0.11 -0.10 -0.09 -0.08 -0.07 -0.06 -0.05 -0.04 -0.03 -0.02 -0.01 0.00 0.01 0.02 0.03 0.04 0.05 0.06 0.07 0.08 0.09 0.10 0.11 0.12 0.13 0.14 0.15]  f_susp_dzdot_bp=[-0.15 -0.14 -0.13 -0.12 -0.11 -0.10 -0.09 -0.08 -0.07 -0.06 -0.05 -0.04 -0.03 -0.02 -0.01 0.00 0.01 0.02 0.03 0.04 0.05 0.06 0.07 0.08 0.09 0.10 0.11 0.12 0.13 0.14 0.15]  f_susp_fmz=zeros(31,31,61,2,4)  f_susp_geom=zeros(31,61,2,3)  f_susp_strgdelta_bp=[-30,-29,-28,-27,-26,-25,-24,-23,-22,-21,-20,-19,-18,-17,-16,-15,-14,-13,-12,-11,-10,-9,-8,-7,-6,-5,-4,-3,-2,-1,0,1,2,3,4,5,6,7,8,9,10,11,12,13,14,15,16,17,18,19,20,21,22,23,24,25,26,27,28,29,30]  AntiSwayR=0.2  AntiSwayNtrlAng=0.5236  AntiSwayTrsK=5.7296e+03
  Matrix Concatenate : Concatenate  NumInputs=4  Mode=Multidimensional array  ConcatenateDimension=2
  Matrix Concatenate1 : Concatenate  NumInputs=4  Mode=Multidimensional array  ConcatenateDimension=2
  Reshape : Reshape  OutputDimensionality=Row vector (2-D)
  Reshape1 : Reshape  OutputDimensionality=Row vector (2-D)
  Selector : Selector  InputPortWidth=4  IndexOptions=Index vector (dialog)  Indices=[1 2]  OutputSizes=1
  Tire Radius : Constant  Value=[tireRadius tireRadius tireRadius tireRadius]
  Transpose : Math  Operator=transpose
  Transpose1 : Math  Operator=transpose
  Vector Concatenate : Concatenate  NumInputs=4
  Vector Concatenate1 : Concatenate  NumInputs=4
  Info : Outport
  VehF : Outport  Port=2
  VehM : Outport  Port=3
  WhlF : Outport  Port=4
  WhlAng : Outport  Port=5
  WhlV : Outport  Port=6
  wires:
  Matrix Concatenate1/1 -> Independent Suspension - Double Wishbone/8
  Independent Suspension - Double Wishbone/4 -> WhlF/1
  Independent Suspension - Double Wishbone/1 -> Info/1
  Selector/1 -> Independent Suspension - Double Wishbone/9
  Tire Radius/1 -> Independent Suspension - Double Wishbone/2
  WhlM/1 -> Independent Suspension - Double Wishbone/6
  Matrix Concatenate/1 -> Independent Suspension - Double Wishbone/7
  Independent Suspension - Double Wishbone/5 -> WhlV/1
  Independent Suspension - Double Wishbone/3 -> VehM/1
  Independent Suspension - Double Wishbone/2 -> Display/1, VehF/1
  Independent Suspension - Double Wishbone/6 -> WhlAng/1
  WhlFy [4,1]/1 -> Transpose/1
  WhlFx [4,1]/1 -> Transpose1/1
  WhlAng [1,4]/1 -> Selector/1
  Transpose/1 -> Independent Suspension - Double Wishbone/5
  Transpose1/1 -> Independent Suspension - Double Wishbone/4
  Bus Selector/1 -> Add Constant/1  "<z>"
  Bus Selector/2 -> Add Constant1/1  "<z>"
  Bus Selector/3 -> Add Constant2/1  "<z>"
  Bus Selector/4 -> Add Constant3/1  "<z>"
  Vector Concatenate/1 -> Display1/1, Reshape/1
  Reshape/1 -> Independent Suspension - Double Wishbone/1
  Vector Concatenate1/1 -> Reshape1/1
  VehInfo/1 -> Bus Selector/1, Bus Selector8/1, Bus Selector9/1, Bus Selector7/1, Bus Selector6/1, Bus Selector5/1, Bus Selector4/1, Bus Selector3/1, Bus Selector2/1, Bus Selector1/1
  Add Constant/1 -> Vector Concatenate/1
  Add Constant1/1 -> Vector Concatenate/2
  Add Constant2/1 -> Vector Concatenate/3
  Add Constant3/1 -> Vector Concatenate/4
  Bus Selector2/1 -> Bus Creator1/1  "<X>"
  Bus Selector2/2 -> Bus Creator1/2  "<Y>"
  Bus Selector2/3 -> Bus Creator1/3  "<Z>"
  Bus Selector3/2 -> Bus Creator2/2  "<Y>"
  Bus Selector3/1 -> Bus Creator2/1  "<X>"
  Bus Selector3/3 -> Bus Creator2/3  "<Z>"
  Bus Selector4/1 -> Bus Creator3/1  "<X>"
  Bus Selector4/2 -> Bus Creator3/2  "<Y>"
  Bus Selector4/3 -> Bus Creator3/3  "<Z>"
  Bus Selector5/1 -> Bus Creator4/1  "<X>"
  Bus Selector5/2 -> Bus Creator4/2  "<Y>"
  Bus Selector5/3 -> Bus Creator4/3  "<Z>"
  Bus Creator4/1 -> Matrix Concatenate/4
  Bus Creator3/1 -> Matrix Concatenate/3
  Bus Creator2/1 -> Matrix Concatenate/2
  Bus Creator1/1 -> Matrix Concatenate/1
  Bus Selector6/1 -> Bus Creator/1  "<Xdot>"
  Bus Selector6/2 -> Bus Creator/2  "<Ydot>"
  Bus Selector6/3 -> Bus Creator/3  "<Zdot>"
  Bus Selector7/2 -> Bus Creator5/2  "<Ydot>"
  Bus Selector7/1 -> Bus Creator5/1  "<Xdot>"
  Bus Selector7/3 -> Bus Creator5/3  "<Zdot>"
  Bus Selector8/1 -> Bus Creator6/1  "<Xdot>"
  Bus Selector8/2 -> Bus Creator6/2  "<Ydot>"
  Bus Selector8/3 -> Bus Creator6/3  "<Zdot>"
  Bus Selector9/1 -> Bus Creator7/1  "<Xdot>"
  Bus Selector9/2 -> Bus Creator7/2  "<Ydot>"
  Bus Selector9/3 -> Bus Creator7/3  "<Zdot>"
  Bus Creator/1 -> Matrix Concatenate1/1
  Bus Creator5/1 -> Matrix Concatenate1/2
  Bus Creator6/1 -> Matrix Concatenate1/3
  Bus Creator7/1 -> Matrix Concatenate1/4
  Bus Selector1/1 -> Gain/1  "<Zdot>"
  Bus Selector1/2 -> Gain1/1  "<Zdot>"
  Bus Selector1/3 -> Gain2/1  "<Zdot>"
  Bus Selector1/4 -> Gain3/1  "<Zdot>"
  Reshape1/1 -> Independent Suspension - Double Wishbone/3
  Gain/1 -> Vector Concatenate1/1
  Gain1/1 -> Vector Concatenate1/2
  Gain2/1 -> Vector Concatenate1/3
  Gain3/1 -> Vector Concatenate1/4

== system Model/Vehicle Information ==
  0 : Constant  Value=[zeros(1,4)]  VectorParams1D=off
  Bus Creator : BusCreator  Inputs=4
  Bus Creator1 : BusCreator  Inputs=4
  Camber : Constant  Value=camber
  Gain : Gain  Gain=-1
  Gain1 : Gain  Gain=-1
  Lambda_mux : Constant  Value=lammux
  Lambda_muy : Constant  Value=lammuy
  Reshape : Reshape  OutputDimensionality=Row vector (2-D)
  Reshape1 : Reshape  OutputDimensionality=Row vector (2-D)
  Tire Pressure : Constant  Value=tirePressure
  Vector Concatenate : Concatenate  NumInputs=5  Mode=Multidimensional array
  Vector Concatenate1 : Concatenate  NumInputs=4
  Vector Concatenate2 : Concatenate  NumInputs=4
  ones : Constant  Value=[ones(23,4)]  VectorParams1D=off
  ones2 : Constant  Value=ones(1,4)  VectorParams1D=off
  Camber [1,4] : Outport
  Tire Pressure [1,4] : Outport  Port=2
  Scaling Factors [4,27] : Outport  Port=3
  wires:
  Camber/1 -> Bus Creator/4, Gain1/1, Bus Creator/2, Gain/1
  Gain/1 -> Bus Creator/1
  Gain1/1 -> Bus Creator/3
  Bus Creator/1 -> Camber [1,4]/1
  Tire Pressure/1 -> Bus Creator1/4, Bus Creator1/3, Bus Creator1/2, Bus Creator1/1
  Bus Creator1/1 -> Tire Pressure [1,4]/1
  Lambda_muy/1 -> Vector Concatenate1/3, Vector Concatenate1/4, Vector Concatenate1/2, Vector Concatenate1/1
  Lambda_mux/1 -> Vector Concatenate2/4, Vector Concatenate2/3, Vector Concatenate2/2, Vector Concatenate2/1
  ones/1 -> Vector Concatenate/5
  Vector Concatenate2/1 -> Reshape/1
  ones2/1 -> Vector Concatenate/1  "lambda_Fz0"
  0/1 -> Vector Concatenate/4  "lamda_mu_V"
  Vector Concatenate/1 -> Scaling Factors [4,27]/1
  Vector Concatenate1/1 -> Reshape1/1
  Reshape/1 -> Vector Concatenate/2
  Reshape1/1 -> Vector Concatenate/3

== system Model/Vehicle Velocity to Wheel Velocity Vectors ==
  VehVel [1,3] : Inport
  WhlAng [1,4] : Inport  Port=2
  Selector : Selector  InputPortWidth=3  IndexOptions=Index vector (dialog)  Indices=[1 2]  OutputSizes=1
  Vehicle Velocity to Wheel Velocity Vectors : MATLAB Function  TreatAsAtomicUnit=on
  Vx : Outport
  Vy : Outport  Port=2
  wires:
  VehVel [1,3]/1 -> Selector/1
  Selector/1 -> Vehicle Velocity to Wheel Velocity Vectors/2(vehVel)
  Vehicle Velocity to Wheel Velocity Vectors/2(Vy) -> Vy/1
  WhlAng [1,4]/1 -> Vehicle Velocity to Wheel Velocity Vectors/1(whlAng)
  Vehicle Velocity to Wheel Velocity Vectors/1(Vx) -> Vx/1

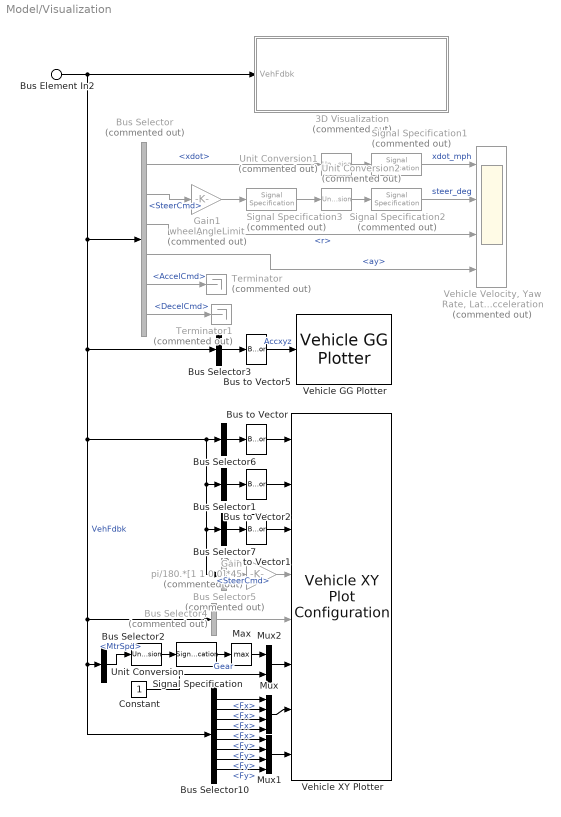
== system Model/Visualization ==
  Bus Element In2 : Inport  PortName=VehFdbk
  3D Visualization : Subsystem  Commented=on  Variant=on  VariantControl=Choice  mask(3D Visualization Setup){engine3D=Disabled, conesOn=off, annotOn=off, InitialPos=[ VEH.InitialLongPosition, VEH.InitialLatPosition, VEH.InitialVertPosition ], InitialRot=[VEH.InitialRollAngle VEH.InitialPitchAngle VEH.InitialYawAngle], Ts=Ts}
      mask prompts: engine3D "Visualization Mode:"; conesOn "Include cones"; annotOn "Include annotations"; InitialPos "shared_sim3dblks:sim3dblkVehicleWithGroundFollowingVDBS:blkPrm_InitialPos"; InitialRot "shared_sim3dblks:sim3dblkVehicleWithGroundFollowingVDBS:blkPrm_InitialRotSAE"; Ts "shared_sim3dblks:sim3dblkConfig:Ts"
      mask help: This is an example specific block designed to only work with vydnblksskidpad.slx. It is used in conjuction with the vehicle subystem to provide options for the 3D game engine visualization (requires Simulink 3D Animation).
      mask init:
      | visType = get_param(gcb,"engine3D");
      | switch visType
      |     case "Disabled"
      |         autoblksenableparameters(gcb, [],{'conesOn';'annotOn'},[],[],true);
      |         set_param([bdroot '/Formula Student Vehicle'],'vehType','Simulink Physics')
      |     case "Enabled - Ground Following Vehicle"
      |         set_param([bdroot '/Formula Student Vehicle'],'vehType','Simulink Physics')
      |         autoblksenableparameters(gcb, {'conesOn';'annotOn'},[],[],[],true);
      |     case "Enabled - Game Physics Vehicle"
      |         set_param([bdroot '/Formula Student Vehicle'],'vehType','Game Engine Physics')
      |         autoblksenableparameters(gcb, {'conesOn';'annotOn'},[],[],[],true);
      | end
      settings: AttributesFormatString=%<engine3D>
      mask TypeOptions engine3D: Disabled | Enabled - Simulink 3D Vehicle | Enabled - Game Physics Vehicle
      mask Callback engine3D:
      | if strcmp(get_param(gcb,"engine3D"),"Disabled")
      |     autoblksenableparameters(gcb, [],{'conesOn';'annotOn'},[],[],true);
      | else
      |     autoblksenableparameters(gcb, {'conesOn';'annotOn'},[],[],[],true);
      | end
      mask DialogControl InitialPos Prompt: Initial position [X, Y, Z], InitialPos [m]:
      mask DialogControl InitialRot Prompt: Initial rotation [Roll, Pitch, Yaw], InitialRot [rad]:
      mask DialogControl Ts Prompt: Sample time:
  Bus Selector : BusSelector  Commented=on  OutputSignals=VehFdbk.BdyFrm.Cg.Vel.xdot,Driver.SteerCmd,VehFdbk.BdyFrm.Cg.AngVel.r,VehFdbk.BdyFrm.Cg.Acc.ay,Driver.AccelCmd,Driver.DecelCmd
  Bus Selector1 : BusSelector  OutputSignals=VehFdbk.InertFrm.Cg.Ang.phi,VehFdbk.InertFrm.Cg.Ang.theta,VehFdbk.InertFrm.Cg.Ang.psi  OutputAsBus=on
  Bus Selector10 : BusSelector  OutputSignals=VehFdbk.BdyFrm.Forces.Tires.FrntTires.Lft.Fx,VehFdbk.BdyFrm.Forces.Tires.FrntTires.Rght.Fx,VehFdbk.BdyFrm.Forces.Tires.RearTires.Lft.Fx,VehFdbk.BdyFrm.Forces.Tires.RearTires.Rght.Fx,VehFdbk.BdyFrm.Forces.Tires.FrntTires.Lft.Fy,VehFdbk.BdyFrm.Forces.Tires.FrntTires.Rght.Fy,VehFdbk.BdyFrm.Forces.Tires.RearTires.Lft.Fy,VehFdbk.BdyFrm.Forces.Tires.RearTires.Rght.Fy
  Bus Selector2 : BusSelector  OutputSignals=VehFdbk.Mtr.MtrSpd
  Bus Selector3 : BusSelector  OutputSignals=VehFdbk.BdyFrm.Cg.Acc.ax,VehFdbk.BdyFrm.Cg.Acc.ay,VehFdbk.BdyFrm.Cg.Acc.az  OutputAsBus=on
  Bus Selector4 : BusSelector  Commented=on  OutputSignals=Driver.Ref  OutputAsBus=on
  Bus Selector5 : BusSelector  Commented=on  OutputSignals=Driver.SteerCmd
  Bus Selector6 : BusSelector  OutputSignals=VehFdbk.InertFrm.Cg.Disp.X,VehFdbk.InertFrm.Cg.Disp.Y,VehFdbk.InertFrm.Cg.Disp.Z  OutputAsBus=on
  Bus Selector7 : BusSelector  OutputSignals=VehFdbk.InertFrm.Cg.Vel.Xdot,VehFdbk.InertFrm.Cg.Vel.Ydot,VehFdbk.InertFrm.Cg.Vel.Zdot  OutputAsBus=on
  Bus to Vector{,1..2,5} (4 alike) : BusToVector
  Constant : Constant
  Gain : Gain  Commented=on  Gain=pi/180.*[1 1 0 0]*45
  Gain1 : Gain  Commented=on  Gain=wheelAngleLimit
  Max : MinMax  Function=max  ZeroCross=off
  Mux : Mux
  Mux1 : Mux
  Mux2 : Mux  Inputs=2
  Signal Specification : SignalSpecification  Unit=rad/s
  Signal Specification1 : SignalSpecification  Commented=on  Unit=mph
  Signal Specification2 : SignalSpecification  Commented=on  Unit=deg
  Signal Specification3 : SignalSpecification  Commented=on  Unit=rad
  Terminator : Terminator  Commented=on
  Terminator1 : Terminator  Commented=on
  Unit Conversion : UnitConversion
  Unit Conversion1 : UnitConversion  Commented=on
  Unit Conversion2 : UnitConversion  Commented=on
  Vehicle GG Plotter : vehdynlibviscommon/Vehicle GG Plotter  axesType=+z down, inertial  gScale=2  pltDT=.1
  "Vehicle Velocity, Yaw Rate, Lateral Acceleration" : Scope  Commented=on  NumInputPorts=4
  Vehicle XY Plotter : vehdynlibviscommon/Vehicle XY Plot Configuration  extRef=on  extStats=on  extTireF=on  a=cgToFrontAxle  b=cgToRearAxle  w=trackWidth  figBorder=10  bufferSize=2048  velNorm=10  tireFNorm=1000  pltDT=.2
  wires:
  Bus Selector7/1 -> Bus to Vector1/1
  Bus to Vector/1 -> Vehicle XY Plotter/1
  Bus Selector6/1 -> Bus to Vector/1
  Bus to Vector1/1 -> Vehicle XY Plotter/3
  Bus Selector1/1 -> Bus to Vector2/1
  Bus Element In2/1 -> 3D Visualization/1(VehFdbk), Bus Selector3/1, Bus Selector10/1, Bus Selector2/1, Bus Selector4/1, Bus Selector5/1, Bus Selector7/1, Bus Selector1/1, Bus Selector6/1, Bus Selector/1  "VehFdbk"
  Bus to Vector2/1 -> Vehicle XY Plotter/2
  Bus Selector5/1 -> Gain/1  "<SteerCmd>"
  Unit Conversion1/1 -> Signal Specification1/1
  Bus Selector/4 -> "Vehicle Velocity, Yaw Rate, Lateral Acceleration"/4  "<ay>"
  Bus Selector/1 -> Unit Conversion1/1  "<xdot>"
  Signal Specification1/1 -> "Vehicle Velocity, Yaw Rate, Lateral Acceleration"/1  "xdot_mph"
  Bus Selector/3 -> "Vehicle Velocity, Yaw Rate, Lateral Acceleration"/3  "<r>"
  Bus Selector4/1 -> Vehicle XY Plotter/5
  Gain/1 -> Vehicle XY Plotter/4
  Mux2/1 -> Vehicle XY Plotter/6
  Constant/1 -> Mux2/2  "Gear"
  Bus Selector/2 -> Gain1/1  "<SteerCmd>"
  Unit Conversion2/1 -> Signal Specification2/1
  Signal Specification2/1 -> "Vehicle Velocity, Yaw Rate, Lateral Acceleration"/2  "steer_deg"
  Bus to Vector5/1 -> Vehicle GG Plotter/1  "Accxyz"
  Bus Selector3/1 -> Bus to Vector5/1
  Mux/1 -> Vehicle XY Plotter/7
  Mux1/1 -> Vehicle XY Plotter/8
  Bus Selector10/1 -> Mux/1  "<Fx>"
  Bus Selector10/2 -> Mux/2  "<Fx>"
  Bus Selector10/3 -> Mux/3  "<Fx>"
  Bus Selector10/4 -> Mux/4  "<Fx>"
  Bus Selector10/5 -> Mux1/1  "<Fy>"
  Bus Selector10/6 -> Mux1/2  "<Fy>"
  Bus Selector10/7 -> Mux1/3  "<Fy>"
  Bus Selector10/8 -> Mux1/4  "<Fy>"
  Gain1/1 -> Signal Specification3/1
  Signal Specification3/1 -> Unit Conversion2/1
  Unit Conversion/1 -> Signal Specification/1
  Bus Selector2/1 -> Unit Conversion/1  "<MtrSpd>"
  Signal Specification/1 -> Max/1
  Bus Selector/5 -> Terminator/1  "<AccelCmd>"
  Bus Selector/6 -> Terminator1/1  "<DecelCmd>"
  Max/1 -> Mux2/1

== system Model/Visualization/3D Visualization ==
  VehFdbk : Inport
  Disabled : Subsystem  VariantControl=engine3D==1
  Enabled : Subsystem  VariantControl=engine3D~=1

== system Model/Visualization/3D Visualization/Disabled ==

== system Model/Visualization/3D Visualization/Enabled ==
  VehFdbk : Inport
  3D Visualization : Subsystem  Variant=on  VariantControl=Choice
  Cones : Subsystem  Variant=on  VariantControl=Choice
  wires:
  VehFdbk/1 -> 3D Visualization/1(VehFdbk)
